simulink subsystem "SWs"  (R2025b)
settings: Solver=VariableStepAuto  StartTime=0.0  StopTime=10.0  RelTol=1e-3
settings Model: Creator=JesseJabezArendse  LastModifiedBy=JesseJabezArendse
settings RTWCC: GPUComputeCapability=3.5

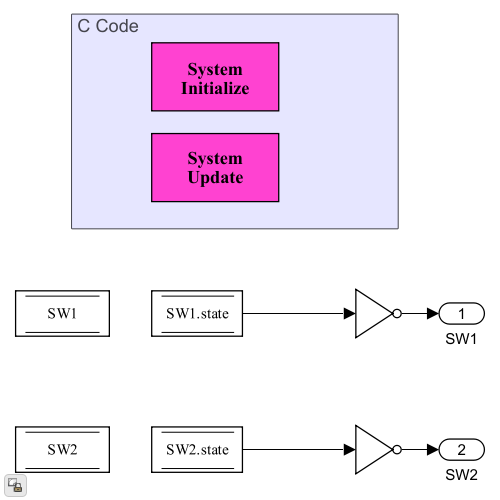
[thumbnail: Simulink's stored preview of the top-level diagram]
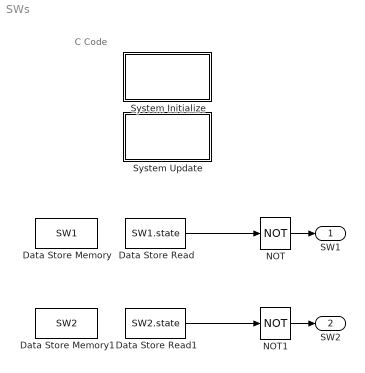
== system SWs ==
  note: C Code
  Data Store Memory : DataStoreMemory  DataStoreName=SW1  WriteAfterWriteMsg=warning  ShowAdditionalParam=off  OutDataTypeStr=Bus: SW_t
  Data Store Memory1 : DataStoreMemory  DataStoreName=SW2  WriteAfterWriteMsg=warning  ShowAdditionalParam=off  OutDataTypeStr=Bus: SW_t
  Data Store Read : DataStoreRead  DataStoreName=SW1  DataStoreElements=SW1.state  IndexOptions=Index vector (dialog)  Indices=1  OutputSizes=1
  Data Store Read1 : DataStoreRead  DataStoreName=SW2  DataStoreElements=SW2.state  IndexOptions=Index vector (dialog)  Indices=1  OutputSizes=1
  NOT : Logic  Operator=NOT  IconShape=distinctive  AllPortsSameDT=off  OutDataTypeStr=boolean
  NOT1 : Logic  Operator=NOT  IconShape=distinctive  AllPortsSameDT=off  OutDataTypeStr=boolean
  System Initialize : Subsystem  mask(System Initialize){ShowInLibBrowser=0}
      mask prompts: ShowInLibBrowser "Simulink:masks:CustCodeMaskParam1_MP"
      settings: CopyFcn=cccopyfcn(gcb)  OpenFcn=ccopenfcn('System Initialize Function')
      mask Help: eval('feval(''rtwprivate'',''rtwhelpview'',''rtw_sys_initialize_block'')');
      mask Display: disp('System\nInitialize');
  System Update : Subsystem  mask(System Update){ShowInLibBrowser=0}
      mask prompts: ShowInLibBrowser "Simulink:masks:CustCodeMaskParam1_MP"
      settings: CopyFcn=cccopyfcn(gcb)  OpenFcn=ccopenfcn('System Update Function')
      mask Help: eval('feval(''rtwprivate'',''rtwhelpview'',''rtw_sys_update_block'')');
      mask Display: disp('System\nUpdate');
  SW1 : Outport
  SW2 : Outport  Port=2
  wires:
  NOT/1 -> SW1/1
  NOT1/1 -> SW2/1
  Data Store Read/1 -> NOT/1
  Data Store Read1/1 -> NOT1/1

== system SWs/System Initialize ==

== system SWs/System Update ==
